simulink model "BE_simu2"  (R2022b)
settings: Solver=VariableStepAuto  StartTime=0.0  StopTime=10  RelTol=1e-3
settings Model: Creator=antoi  LastModifiedBy=guilhermepifferchristo
settings SolverCC: AlgebraicLoopSolver=TrustRegion
settings DebuggingCC: UnconnectedInputMsg=warning  UnconnectedOutputMsg=warning  UnconnectedLineMsg=warning  SFMachineParentedDataDiag=warning  UnderSpecifiedDimensionMsg=error  ArithmeticOperatorsInVariantConditions=warning
settings ModelReferenceCC: EnableRefExpFcnMdlSchedulingChecks=on
settings SFSimCC: CustomCodeUndefinedFunction=UseInterfaceOnly

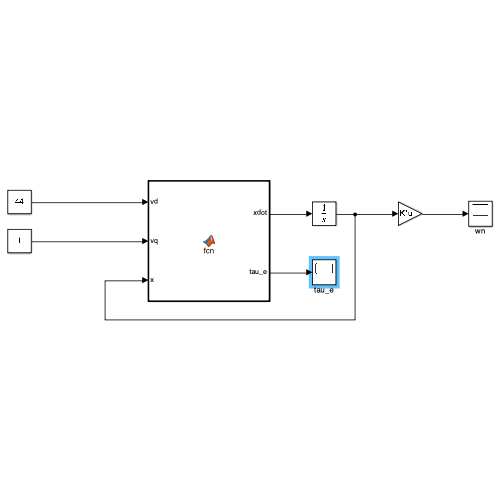
[thumbnail: Simulink's stored preview of the top-level diagram]
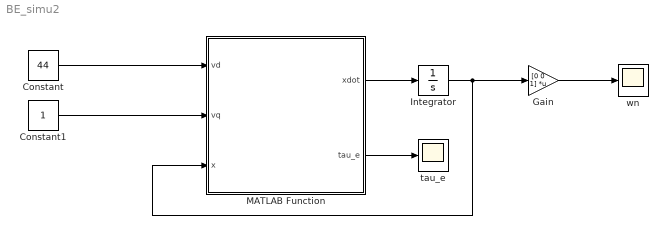
== system BE_simu2 ==
  Constant : Constant  Value=44
  Constant1 : Constant
  Gain : Gain  Gain=[0 0 1]  Multiplication=Matrix(K*u)
  Integrator : Integrator  InitialCondition=[0 ;0 ;0]
  MATLAB Function : MATLAB Function  TreatAsAtomicUnit=on
  tau_e : Scope
  wn : Scope
  wires:
  Constant/1 -> MATLAB Function/1(vd)
  MATLAB Function/1(xdot) -> Integrator/1
  MATLAB Function/2(tau_e) -> tau_e/1
  Integrator/1 -> Gain/1, MATLAB Function/3(x)
  Gain/1 -> wn/1
  Constant1/1 -> MATLAB Function/2(vq)

== matlab function BE_simu2/MATLAB Function ==
  data: vd input; xdot output; vq input; x input; tau_e output
function [xdot,tau_e]= fcn(vd, vq, x)
    Rs = 0.124 ;
    Ls = 0.0021 ;
    lambm = 0.0744 ;
    Np = 52 ;
    M = 92 ;
    Rw = 0.33 ;
    Jt = M*Rw*Rw ;
    Ca = 0.18 ;
    s = 0.05 ;
    tau_c = 0 ;
    g = 9.81 ;
    
    tau_e = (3*Np*lambm/4) * x(2) ;
    tau_load = M*g*s*Rw + Ca*(Rw^3)*(x(3)^2) ;
    
    xdot1 =  -(Rs/Ls)*x(1) + (Np/2)*x(2)*x(3) + vd/Ls ;
    xdot2 = -(Rs/Ls)*x(2) - (Np/2)*x(1)*x(3) - (Np/2)*(lambm/Ls)*x(3) + vq/Ls ; 
    xdot3 = (1/Jt)*(tau_e - tau_load + tau_c)  ;
    xdot=[xdot1 ; xdot2 ; xdot3] ;
end
